simulink model "robot_arm"  (R2024a)
settings: Solver=VariableStepAuto  StartTime=0.0  StopTime=Tsim  RelTol=1e-3
values from neighbouring files (symbols this model uses):
  mag = 0.1    [one_link_robot_arm_integral.m]    (also in robot_arm_pi.m = 1; robot_arm_state_feedback.m; robust_state_feedback.m = 1)
  Ts = 0.1    [one_link_robot_arm_integral.m]    (also in robot_arm_pi.m; robot_arm_state_feedback.m)
  x0 = (2*mx0).*rand(5,1)-mx0    [one_link_robot_arm_integral.m]    (also in robot_arm_pi.m = (2*mag).*rand(5,1)-mag; robot_arm_state_feedback.m = (2*mx0).*rand(n,1)-mx0)
settings Model: Creator=pietrotesi  LastModifiedBy=watch
settings SolverCC: AlgebraicLoopSolver=TrustRegion
settings DataIOCC: ReturnWorkspaceOutputs=off
settings DebuggingCC: UnconnectedInputMsg=warning  UnconnectedOutputMsg=warning  UnconnectedLineMsg=warning
settings ModelReferenceCC: EnableRefExpFcnMdlSchedulingChecks=on
settings RTWCC: GPUComputeCapability=3.5  DLArmComputeVersion=19.05

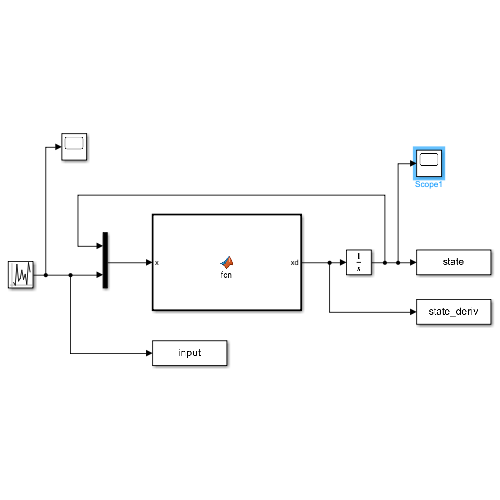
[thumbnail: Simulink's stored preview of the top-level diagram]
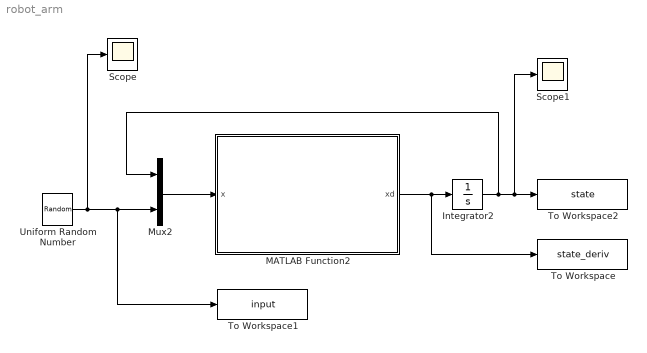
== system robot_arm ==
  Integrator2 : Integrator  InitialCondition=x0
  MATLAB Function2 : MATLAB Function  TreatAsAtomicUnit=on
  Mux2 : Mux  Inputs=2
  Scope : Scope
  Scope1 : Scope
  To Workspace : ToWorkspace  VariableName=state_deriv  SaveFormat=Structure With Time  SampleTime=Ts
  To Workspace1 : ToWorkspace  VariableName=input  SaveFormat=Structure With Time  SampleTime=Ts
  To Workspace2 : ToWorkspace  VariableName=state  SaveFormat=Structure With Time  SampleTime=Ts
  Uniform Random Number : UniformRandomNumber  Minimum=-mag  Maximum=mag  SampleTime=Ts
  wires:
  Mux2/1 -> MATLAB Function2/1(x)
  MATLAB Function2/1(xd) -> To Workspace/1, Integrator2/1
  Uniform Random Number/1 -> Scope/1, To Workspace1/1, Mux2/2
  Integrator2/1 -> Mux2/1, Scope1/1, To Workspace2/1

== matlab function robot_arm/MATLAB Function2 ==
  data: x input; xd output
function xd = fcn(x)

x1 = x(1);
u  = x(5);

A = [0 1 0 0; ... % precomputed A matrix
    -2 -0.75 1 0; ...
    0 0 0 1; ...
    -1.3 0 0.66 -0.2];
B = [0; 0; 0; 6.6]; % precomputed B matrix

xd = A*x(1:4) + B*u;
xd(2) = xd(2) -1.96*cos(x1);
